simulink model "q4TH"  (Simulink 5.0)
settings: Solver=ode45  StartTime=0.0  StopTime=10.0  RelTol=1e-3
settings Model: LastModifiedBy=Frank Gloria

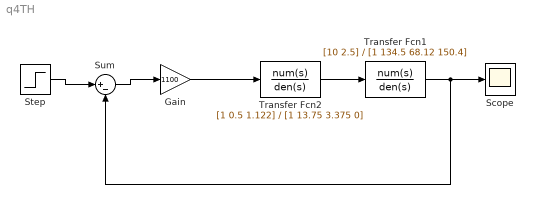
== system q4TH ==
  Gain : Gain  Gain=1100  SaturateOnIntegerOverflow=on
  Scope : Scope
  Step : Step  Time=0  SampleTime=0
  Sum : Sum  Inputs=|+-  SaturateOnIntegerOverflow=on
  Transfer Fcn1 : TransferFcn  Numerator=[10 2.5]  Denominator=[1 134.5 68.12 150.4]
  Transfer Fcn2 : TransferFcn  Numerator=[1 0.5 1.122]  Denominator=[1 13.75 3.375 0]
  wires:
  Step/1 -> Sum/1
  Sum/1 -> Gain/1
  Gain/1 -> Transfer Fcn2/1
  Transfer Fcn2/1 -> Transfer Fcn1/1
  Transfer Fcn1/1 -> Scope/1, Sum/2
